simulink model "MBD_GroupJ_Oxy"  (R2022a)
settings: Solver=VariableStepAuto  StartTime=0.0  StopTime=10.0  RelTol=1e-3
model workspace (MAT data in the model file):
  x = 50
libraries: simulink x9
settings Model: Creator=hp  LastModifiedBy=hp

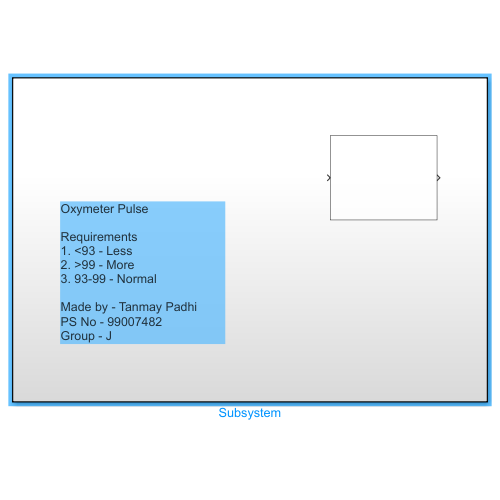
[thumbnail: Simulink's stored preview of the top-level diagram]
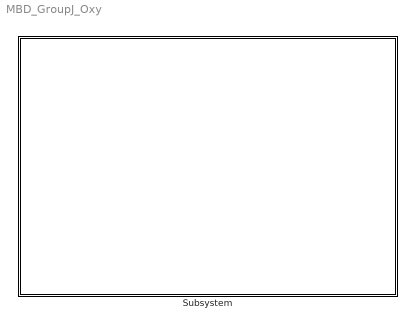
== system MBD_GroupJ_Oxy ==
  Subsystem : Subsystem

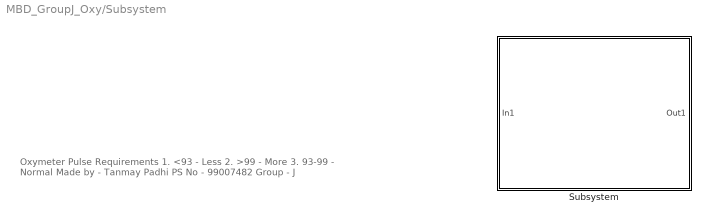
== system MBD_GroupJ_Oxy/Subsystem ==
  note: Oxymeter Pulse
      |
      | Requirements
      | 1. <93 - Less
      | 2. >99 - More
      | 3. 93-99 - Normal
      |
      | Made by - Tanmay Padhi
      | PS No - 99007482
      | Group - J
  Subsystem : Subsystem

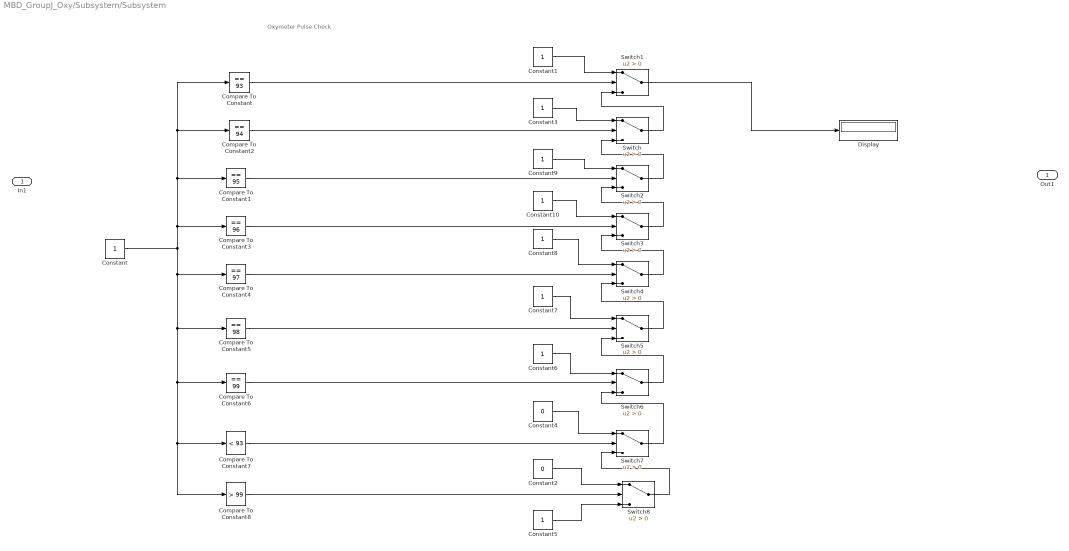
== system MBD_GroupJ_Oxy/Subsystem/Subsystem ==
  note: Oxymeter Pulse Check
  In1 : Inport
  Compare To Constant : simulink/Logic and Bit Operations/Compare To Constant  relop===  const=93  OutDataTypeStr=boolean
  Compare To Constant1 : simulink/Logic and Bit Operations/Compare To Constant  relop===  const=95  OutDataTypeStr=boolean
  Compare To Constant2 : simulink/Logic and Bit Operations/Compare To Constant  relop===  const=94  OutDataTypeStr=boolean
  Compare To Constant3 : simulink/Logic and Bit Operations/Compare To Constant  relop===  const=96  OutDataTypeStr=boolean
  Compare To Constant4 : simulink/Logic and Bit Operations/Compare To Constant  relop===  const=97  OutDataTypeStr=boolean
  Compare To Constant5 : simulink/Logic and Bit Operations/Compare To Constant  relop===  const=98  OutDataTypeStr=boolean
  Compare To Constant6 : simulink/Logic and Bit Operations/Compare To Constant  relop===  const=99  OutDataTypeStr=boolean
  Compare To Constant7 : simulink/Logic and Bit Operations/Compare To Constant  relop=<  const=93  OutDataTypeStr=boolean
  Compare To Constant8 : simulink/Logic and Bit Operations/Compare To Constant  relop=>  const=99  OutDataTypeStr=boolean
  Constant{,1,3,5..10} (9 alike) : Constant
  Constant2 : Constant  Value=0
  Constant4 : Constant  Value=0
  Display : Display
  Switch{,1..8} (9 alike) : Switch  Criteria=u2 > Threshold  SaturateOnIntegerOverflow=off  InputSameDT=off
  Out1 : Outport
  wires:
  Switch/1 -> Switch1/3
  Constant6/1 -> Switch6/1
  Switch8/1 -> Switch7/3
  Constant4/1 -> Switch7/1
  Compare To Constant7/1 -> Switch7/2
  Constant/1 -> Compare To Constant4/1, Compare To Constant5/1, Compare To Constant8/1, Compare To Constant7/1, Compare To Constant6/1, Compare To Constant2/1, Compare To Constant/1, Compare To Constant1/1, Compare To Constant3/1
  Switch6/1 -> Switch5/3
  Switch2/1 -> Switch/3
  Constant9/1 -> Switch2/1
  Compare To Constant8/1 -> Switch8/2
  Compare To Constant4/1 -> Switch4/2
  Constant5/1 -> Switch8/3
  Compare To Constant1/1 -> Switch2/2
  Compare To Constant5/1 -> Switch5/2
  Constant3/1 -> Switch/1
  Compare To Constant/1 -> Switch1/2
  Constant2/1 -> Switch8/1
  Switch3/1 -> Switch2/3
  Switch4/1 -> Switch3/3
  Compare To Constant3/1 -> Switch3/2
  Switch5/1 -> Switch4/3
  Constant10/1 -> Switch3/1
  Switch1/1 -> Display/1
  Constant8/1 -> Switch4/1
  Constant7/1 -> Switch5/1
  Compare To Constant6/1 -> Switch6/2
  Switch7/1 -> Switch6/3
  Compare To Constant2/1 -> Switch/2
  Constant1/1 -> Switch1/1
